simulink model "fuzzy_pid_feedfowaard"  (Simulink 6.4)
settings: Solver=ode45  StartTime=0.0  StopTime=10.0  RelTol=1e-3
libraries: fuzblock x1
settings Model: LastModifiedBy=Administrator

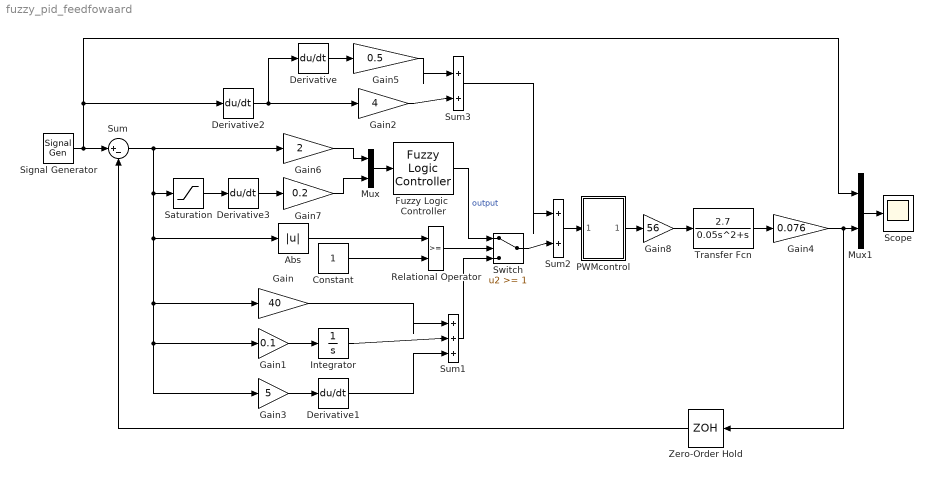
== system fuzzy_pid_feedfowaard ==
  Abs : Abs  SaturateOnIntegerOverflow=on  SampleTime=-1
  Constant : Constant  Value=1  OutDataType=sfix(16)  ConRadixGroup=Use specified scaling  OutScaling=2^0  SampleTime=inf  FramePeriod=inf
  Derivative{,1..3} (4 alike) : Derivative
  Fuzzy Logic  Controller : fuzblock/Fuzzy Logic  Controller  SystemSampleTime=-1  fis=demo1
  Gain : Gain  Gain=40  SaturateOnIntegerOverflow=on
  Gain1 : Gain  Gain=0.1  SaturateOnIntegerOverflow=on
  Gain2 : Gain  Gain=4  SaturateOnIntegerOverflow=on
  Gain3 : Gain  Gain=5  SaturateOnIntegerOverflow=on
  Gain4 : Gain  Gain=0.076  SaturateOnIntegerOverflow=on
  Gain5 : Gain  Gain=0.5  SaturateOnIntegerOverflow=on
  Gain6 : Gain  Gain=2  SaturateOnIntegerOverflow=on
  Gain7 : Gain  Gain=0.2  SaturateOnIntegerOverflow=on
  Gain8 : Gain  Gain=56  SaturateOnIntegerOverflow=on
  Integrator : Integrator
  Mux : Mux  Inputs=2
  Mux1 : Mux  Inputs=2
  PWMcontrol : Subsystem
  Relational Operator : RelationalOperator  InputSameDT=on
  Saturation : Saturate  UpperLimit=10  LowerLimit=-10
  Scope : Scope
      settings: TimeRange=100  YMin=-12  YMax=12  MaxDataPoints=10000
  Signal Generator : SignalGenerator  Amplitude=10  Frequency=10  Units=rad/sec
  Sum : Sum  Inputs=|+-  SaturateOnIntegerOverflow=on  InputSameDT=on
  Sum1 : Sum  Inputs=|+++  SaturateOnIntegerOverflow=on  InputSameDT=on
  Sum2 : Sum  Inputs=|++  SaturateOnIntegerOverflow=on  InputSameDT=on
  Sum3 : Sum  Inputs=|++  SaturateOnIntegerOverflow=on  InputSameDT=on
  Switch : Switch  Threshold=1  SaturateOnIntegerOverflow=on  InputSameDT=on
  Transfer Fcn : TransferFcn  Numerator=[2.7]  Denominator=[0.05 1 0]
  Zero-Order Hold : ZeroOrderHold  Orientation=left  SampleTime=0.0000001
  wires:
  Transfer Fcn/1 -> Gain4/1
  Signal Generator/1 -> Sum/1, Mux1/1, Derivative2/1
  Mux1/1 -> Scope/1
  Gain4/1 -> Mux1/2, Zero-Order Hold/1
  Gain1/1 -> Integrator/1
  Gain3/1 -> Derivative1/1
  Gain/1 -> Sum1/1
  Integrator/1 -> Sum1/2
  Derivative1/1 -> Sum1/3
  Sum2/1 -> PWMcontrol/1(In1)
  Sum/1 -> Gain6/1, Gain/1, Gain3/1, Gain1/1, Abs/1, Saturation/1
  Derivative2/1 -> Gain2/1, Derivative/1
  Derivative/1 -> Gain5/1
  Gain5/1 -> Sum3/1
  Gain2/1 -> Sum3/2
  Sum3/1 -> Sum2/1
  Constant/1 -> Relational Operator/2
  Relational Operator/1 -> Switch/2
  Abs/1 -> Relational Operator/1
  Derivative3/1 -> Gain7/1
  Gain6/1 -> Mux/1
  Mux/1 -> Fuzzy Logic  Controller/1
  Gain7/1 -> Mux/2
  Saturation/1 -> Derivative3/1
  Fuzzy Logic  Controller/1 -> Switch/1  "output"
  Sum1/1 -> Switch/3
  Switch/1 -> Sum2/2
  PWMcontrol/1(Out1) -> Gain8/1
  Gain8/1 -> Transfer Fcn/1
  Zero-Order Hold/1 -> Sum/2

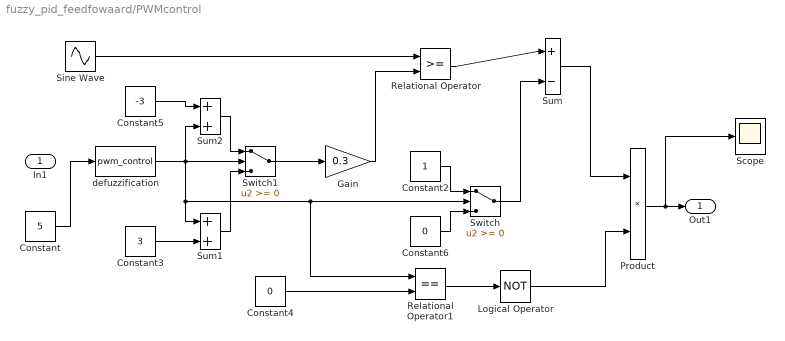
== system fuzzy_pid_feedfowaard/PWMcontrol ==
  In1 : Inport
  Constant : Constant  Value=5  OutDataType=sfix(16)  ConRadixGroup=Use specified scaling  OutScaling=2^0  SampleTime=inf  FramePeriod=inf
  Constant2 : Constant  Value=1  OutDataType=sfix(16)  ConRadixGroup=Use specified scaling  OutScaling=2^0  SampleTime=inf  FramePeriod=inf
  Constant3 : Constant  Value=3  OutDataType=sfix(16)  ConRadixGroup=Use specified scaling  OutScaling=2^0  SampleTime=inf  FramePeriod=inf
  Constant4 : Constant  Value=0  OutDataType=sfix(16)  ConRadixGroup=Use specified scaling  OutScaling=2^0  SampleTime=inf  FramePeriod=inf
  Constant5 : Constant  Value=-3  OutDataType=sfix(16)  ConRadixGroup=Use specified scaling  OutScaling=2^0  SampleTime=inf  FramePeriod=inf
  Constant6 : Constant  Value=0  OutDataType=sfix(16)  ConRadixGroup=Use specified scaling  OutScaling=2^0  SampleTime=inf  FramePeriod=inf
  Gain : Gain  Gain=0.3  SaturateOnIntegerOverflow=on
  Logical Operator : Logic  Operator=NOT  Inputs=1
  Product : Product  SaturateOnIntegerOverflow=on  RndMeth=Zero  InputSameDT=on
  Relational Operator : RelationalOperator  InputSameDT=on
  Relational Operator1 : RelationalOperator  Operator===  InputSameDT=on
  Scope : Scope
      settings: TimeRange=5  YMin=0  YMax=7  MaxDataPoints=10000
  Sine Wave : Sin  Frequency=10000  SampleTime=0
  Sum : Sum  Inputs=|+-  SaturateOnIntegerOverflow=on  InputSameDT=on
  Sum1 : Sum  Inputs=|++  SaturateOnIntegerOverflow=on  InputSameDT=on
  Sum2 : Sum  Inputs=|++  SaturateOnIntegerOverflow=on  InputSameDT=on
  Switch : Switch  SaturateOnIntegerOverflow=on  InputSameDT=on
  Switch1 : Switch  SaturateOnIntegerOverflow=on  InputSameDT=on
  defuzzification : MATLABFcn  MATLABFcn=pwm_control  OutputDimensions=1
  Out1 : Outport
  wires:
  Sum/1 -> Product/1
  Switch/1 -> Sum/2
  Relational Operator/1 -> Sum/1
  Constant5/1 -> Sum2/1
  Sum1/1 -> Switch1/3
  Constant3/1 -> Sum1/2
  Sum2/1 -> Switch1/1
  Constant6/1 -> Switch/3
  Constant2/1 -> Switch/1
  Switch1/1 -> Gain/1
  defuzzification/1 -> Sum1/1, Relational Operator1/1, Switch/2, Sum2/2, Switch1/2
  Logical Operator/1 -> Product/2
  Sine Wave/1 -> Relational Operator/1
  Relational Operator1/1 -> Logical Operator/1
  Constant4/1 -> Relational Operator1/2
  Product/1 -> Out1/1, Scope/1
  Gain/1 -> Relational Operator/2
  Constant/1 -> defuzzification/1
